simulink model "part2_A"  (R2014a)
settings: Solver=ode45  StartTime=0.0  StopTime=10.0  RelTol=1e-3
libraries: slctrlblks x1
settings Model: Creator=gabriellemerritt  LastModifiedBy=gabriellemerritt

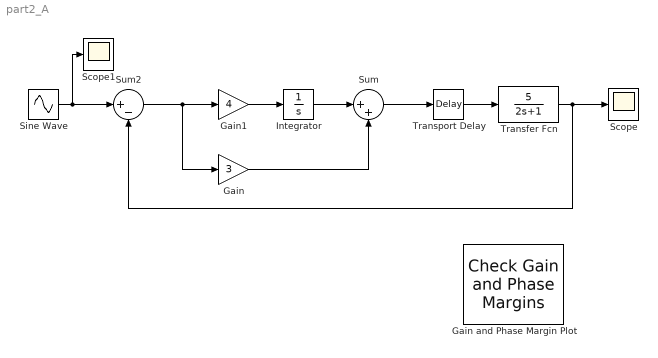
== system part2_A ==
  Gain : Gain  Gain=3
  Gain and Phase Margin Plot : slctrlblks/Model Verification/Check Gain and Phase Margins  InstantiateOnLoad=on  SaveOperatingPoints=off  LinearizationIOs={'/Transfer Fcn', 1, 'out', 'on', '';'/Sum', 1, 'in', 'on', ''}  LinearizeAt=SnapshotTimes  SnapshotTimes=[0]  TriggerType=rising  SampleTime=auto  RateConversionMethod=zoh  PreWarpFreq=10  UseExactDelayModel=off  UseFullBlockNameLabels=off  UseBusSignalLabels=off  enabled=on  stopWhenAssertionFail=off  export=off  ViewDlgPos=[100 106 1027 484]  LaunchViewOnOpen=off  OpenViewOnLoad=off  FrequencyUnits=rad/s  MagnitudeUnits=dB  PhaseUnits=deg  TimeUnits=seconds  EnableMargins=off  GainMargin=[]  PhaseMargin=[]  PlotType=bode  FeedbackSign=-1
      settings: SaveToWorkspace=off  SaveName=sys
  Gain1 : Gain  Gain=4
  Integrator : Integrator
  Scope : Scope
      settings: SaveName=output
  Scope1 : Scope
      settings: SaveName=input
  Sine Wave : Sin  Amplitude=2  SampleTime=0
  Sum : Sum  Inputs=|++
  Sum2 : Sum  Inputs=|+-
  Transfer Fcn : TransferFcn  Numerator=[5]  Denominator=[2 1]
  Transport Delay : TransportDelay  DelayTime=.1
  wires:
  Gain1/1 -> Integrator/1
  Integrator/1 -> Sum/1
  Gain/1 -> Sum/2
  Sum2/1 -> Gain/1, Gain1/1
  Transport Delay/1 -> Transfer Fcn/1
  Transfer Fcn/1 -> Scope/1, Sum2/2
  Sine Wave/1 -> Scope1/1, Sum2/1
  Sum/1 -> Transport Delay/1
